simulink model "booster_compensator"  (R2024b)
settings: Solver=VariableStepAuto  StartTime=0.0  StopTime=Tfin_comp  RelTol=1e-3
values from neighbouring files (symbols this model uses):
  a = pi*r^2    (= 78.5398163397)    [script_project.m]
  Aobs = A-L*C    [script_project.m]
  Bobs = [B L]    [script_project.m]
  Cd = 1.2    [script_project.m]
  Cobs = eye(4)    [script_project.m]
  Dobs = zeros(4, 5)    [script_project.m]
  g = 9.81    [script_project.m]
  h = 70    [script_project.m]
  J = (1/12)*m*(b^2 + h^2)    (= 208333333.333)    [script_project.m]
  K = -place(A, B, desired_poles)    [script_project.m]
  m = 500000    [script_project.m]
  rho = 1.225    [script_project.m]
  u0 = [u1eq u2eq u3eq]'    [script_project.m]
  z0 = [x2eq x2doteq thetaeq thetadoteq]'    [script_project.m]
  z0_comp = z0 + dz0_comp    [script_project.m]
undefined symbols (not defined in the file or in its folder): A, B, C
settings Model: Creator=martinhaugen  LastModifiedBy=martinhaugen

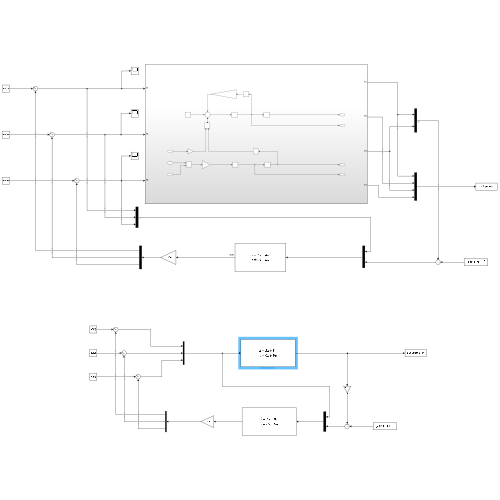
[thumbnail: Simulink's stored preview of the top-level diagram]
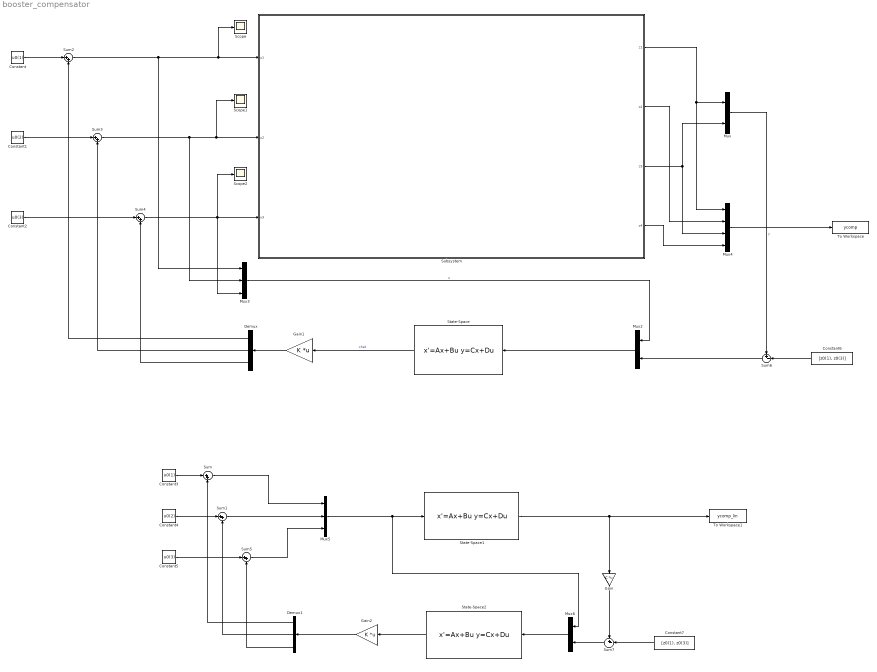
== system booster_compensator ==
  Constant : Constant  Value=u0(1)
  Constant1 : Constant  Value=u0(2)
  Constant2 : Constant  Value=u0(3)
  Constant3 : Constant  Value=u0(1)
  Constant4 : Constant  Value=u0(2)
  Constant5 : Constant  Value=u0(3)
  Constant6 : Constant  Value=[z0(1), z0(3)]
  Constant7 : Constant  Value=[z0(1), z0(3)]
  Demux : Demux  Outputs=3
  Demux1 : Demux  Outputs=3
  Gain : Gain  Gain=C  Multiplication=Matrix(K*u)
  Gain1 : Gain  Gain=K  Multiplication=Matrix(K*u)
  Gain2 : Gain  Gain=K  Multiplication=Matrix(K*u)
  Mux : Mux  Inputs=2
  Mux2 : Mux  Inputs=2
  Mux3 : Mux  Inputs=3
  Mux4 : Mux
  Mux5 : Mux  Inputs=3
  Mux6 : Mux  Inputs=2
  Scope : Scope
  Scope1 : Scope
  Scope2 : Scope
  State-Space : StateSpace  A=Aobs  B=Bobs  C=Cobs  D=Dobs  InitialCondition=z0_comp
  State-Space1 : StateSpace  A=A  B=B  C=eye(4)  D=zeros(4,3)  InitialCondition=z0_comp
  State-Space2 : StateSpace  A=Aobs  B=Bobs  C=Cobs  D=Dobs  InitialCondition=z0_comp
  Subsystem : Subsystem
  Sum{,1..5} (6 alike) : Sum  Inputs=|++
  Sum6 : Sum  Inputs=+-|
  Sum7 : Sum  Inputs=+-|
  To Workspace : ToWorkspace  VariableName=ycomp  SaveFormat=Timeseries  SampleTime=-1
  To Workspace1 : ToWorkspace  VariableName=ycomp_lin  SaveFormat=Timeseries  SampleTime=-1
  wires:
  Subsystem/3(z3) -> Mux4/3, Mux/2
  Subsystem/1(z1) -> Mux/1, Mux4/1
  Mux5/1 -> State-Space1/1, Mux6/1
  Mux6/1 -> State-Space2/1
  Mux4/1 -> To Workspace/1
  State-Space1/1 -> To Workspace1/1, Gain/1
  Subsystem/4(z4) -> Mux4/4
  Mux2/1 -> State-Space/1
  Subsystem/2(z2) -> Mux4/2
  State-Space/1 -> Gain1/1  "xhat"
  Gain1/1 -> Demux/1
  Demux/1 -> Sum2/2
  Constant/1 -> Sum2/1
  Constant1/1 -> Sum3/1
  Constant2/1 -> Sum4/1
  Demux/2 -> Sum3/2
  Demux/3 -> Sum4/2
  Sum2/1 -> Subsystem/1(u1), Scope/1, Mux3/1
  Sum3/1 -> Subsystem/2(u2), Scope1/1, Mux3/2
  Sum4/1 -> Subsystem/3(u3), Mux3/3, Scope2/1
  Mux3/1 -> Mux2/1  "u"
  State-Space2/1 -> Gain2/1
  Gain2/1 -> Demux1/1
  Constant3/1 -> Sum/1
  Constant4/1 -> Sum1/1
  Constant5/1 -> Sum5/1
  Demux1/1 -> Sum/2
  Demux1/2 -> Sum1/2
  Demux1/3 -> Sum5/2
  Sum/1 -> Mux5/1
  Sum1/1 -> Mux5/2
  Sum5/1 -> Mux5/3
  Constant7/1 -> Sum7/2
  Gain/1 -> Sum7/1
  Sum7/1 -> Mux6/2
  Constant6/1 -> Sum6/2
  Sum6/1 -> Mux2/2
  Mux/1 -> Sum6/1  "y"

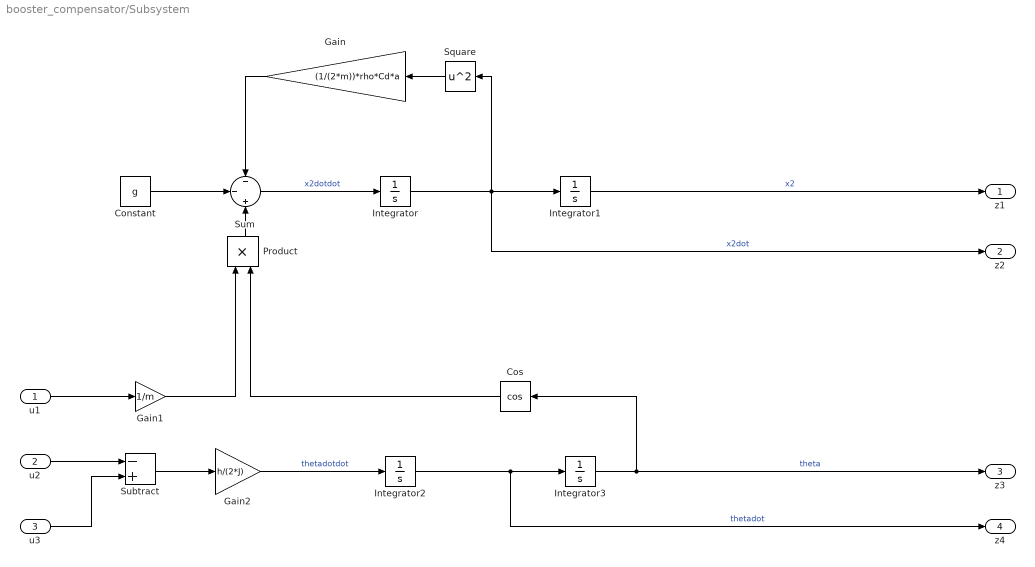
== system booster_compensator/Subsystem ==
  u1 : Inport
  u2 : Inport  Port=2
  u3 : Inport  Port=3
  Constant : Constant  Value=g
  Cos : Trigonometry  Operator=cos
  Gain : Gain  Gain=(1/(2*m))*rho*Cd*a
  Gain1 : Gain  Gain=1/m
  Gain2 : Gain  Gain=h/(2*J)
  Integrator : Integrator  InitialCondition=z0_comp(2)  ContinuousStateAttributes='z2'
  Integrator1 : Integrator  InitialCondition=z0_comp(1)  ContinuousStateAttributes='z1'
  Integrator2 : Integrator  InitialCondition=z0_comp(4)  ContinuousStateAttributes='z4'
  Integrator3 : Integrator  InitialCondition=z0_comp(3)  ContinuousStateAttributes='z3'
  Product : Product
  Square : Math  Operator=square
  Subtract : Sum  Inputs=-+
  Sum : Sum  Inputs=-|-|+
  z1 : Outport
  z2 : Outport  Port=2
  z3 : Outport  Port=3
  z4 : Outport  Port=4
  wires:
  u2/1 -> Subtract/1
  Constant/1 -> Sum/2
  Square/1 -> Gain/1
  Product/1 -> Sum/3
  Subtract/1 -> Gain2/1
  Integrator/1 -> z2/1, Integrator1/1, Square/1  "x2dot"
  Gain2/1 -> Integrator2/1  "thetadotdot"
  Cos/1 -> Product/2
  u3/1 -> Subtract/2
  Integrator2/1 -> z4/1, Integrator3/1  "thetadot"
  u1/1 -> Gain1/1
  Gain/1 -> Sum/1
  Sum/1 -> Integrator/1  "x2dotdot"
  Gain1/1 -> Product/1
  Integrator3/1 -> z3/1, Cos/1  "theta"
  Integrator1/1 -> z1/1  "x2"
